simulink model "StateCharts"  (R2023b)
settings: Solver=VariableStepAuto  StartTime=0.0  StopTime=30  RelTol=1e-3
settings Model: Creator=Hirbod  LastModifiedBy=Hirbod

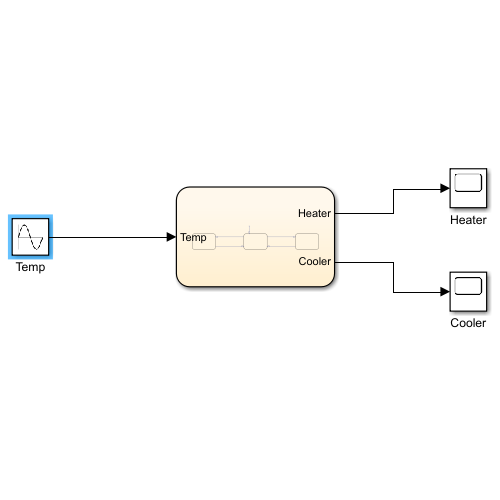
[thumbnail: Simulink's stored preview of the top-level diagram]
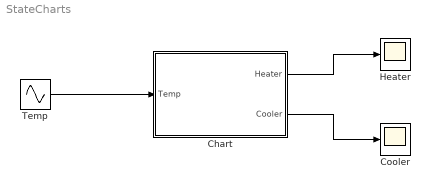
== system StateCharts ==
  Chart : Stateflow chart  TreatAsAtomicUnit=on
  Cooler : Scope
  Heater : Scope
  Temp : Sin  Amplitude=50  SampleTime=0
  wires:
  Temp/1 -> Chart/1(Temp)
  Chart/1(Heater) -> Heater/1
  Chart/2(Cooler) -> Cooler/1

== stateflow chart StateCharts/Chart ==
  state heater_on
    Heater = 1;
    Cooler = 0;
  state initial
    Heater = 0;
    Cooler = 0;
  state cooler_on
    Heater = 0;
    Cooler = 1;
  (default) -> initial
  initial -> heater_on [order 2] : [Temp < 20]
  initial -> cooler_on [order 1] : [Temp > 35]
  heater_on -> initial : [Temp > 25]
  cooler_on -> initial : [Temp < 30]
  data: Temp input; Heater output; Cooler output
